simulink model "MotorCD2"  (Simulink 5.0)
settings: Solver=ode45  StartTime=0.0  StopTime=10.0  RelTol=1e-3
values from neighbouring files (symbols this model uses):
  B = 20    [MasaEjemplo1_valores.m]    (also in VariablesMotorCD.m = 0.01)
  J = 0.02    [VariablesMotorCD.m]
  Kb = 0.11    [VariablesMotorCD.m]
  Ki = 0.11    [VariablesMotorCD.m]
  La = 0.02    [VariablesMotorCD.m]
  Ra = 2    [VariablesMotorCD.m]
settings Model: LastModifiedBy=gaby

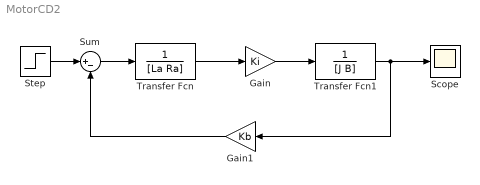
== system MotorCD2 ==
  Gain : Gain  Gain=Ki  SaturateOnIntegerOverflow=on
  Gain1 : Gain  Orientation=left  Gain=Kb  SaturateOnIntegerOverflow=on
  Scope : Scope
  Step : Step  Time=0  After=20  SampleTime=0
  Sum : Sum  Inputs=|+-  SaturateOnIntegerOverflow=on
  Transfer Fcn : TransferFcn  Denominator=[La Ra]
  Transfer Fcn1 : TransferFcn  Denominator=[J B]
  wires:
  Step/1 -> Sum/1
  Sum/1 -> Transfer Fcn/1
  Transfer Fcn/1 -> Gain/1
  Gain/1 -> Transfer Fcn1/1
  Transfer Fcn1/1 -> Gain1/1, Scope/1
  Gain1/1 -> Sum/2
